simulink model "Vodorod_test_VD"  (R2018b)
settings: Solver=VariableStepAuto  StartTime=0.0  StopTime=1.5  RelTol=1e-3
undefined symbols (not defined in the file): C_cond, DiscIntNeverNeededParam, f, L_dros, L_dros_L4, L_dros_L5, R_cond, R_dros_L4, R_dros_L5, Rc, Rv, Um
libraries: powerlib x26, simulink x2, simulink_extras x1
settings Model: Creator=sr1  LastModifiedBy=sr1

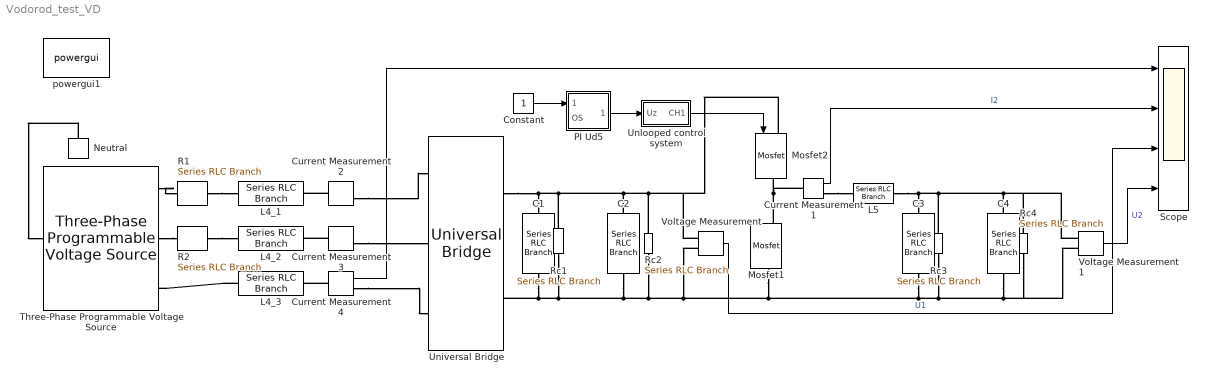
== system Vodorod_test_VD ==
  "C1 " : powerlib/Elements/Series RLC Branch  LConnTagsString=__new0  RConnTagsString=__new0  BranchType=RC  Resistance=R_cond  Inductance=L_dros  SetiL0=off  InitialCurrent=0  Capacitance=C_cond  Setx0=on  InitialVoltage=550  Measurements=None
  C2 : powerlib/Elements/Series RLC Branch  LConnTagsString=__new0  RConnTagsString=__new0  BranchType=RC  Resistance=R_cond  Inductance=L_dros  SetiL0=off  InitialCurrent=0  Capacitance=C_cond  Setx0=on  InitialVoltage=550  Measurements=None
  C3 : powerlib/Elements/Series RLC Branch  LConnTagsString=__new0  RConnTagsString=__new0  BranchType=RC  Resistance=R_cond  Inductance=L_dros  SetiL0=off  InitialCurrent=0  Capacitance=C_cond  Setx0=on  InitialVoltage=0  Measurements=None
  C4 : powerlib/Elements/Series RLC Branch  LConnTagsString=__new0  RConnTagsString=__new0  BranchType=RC  Resistance=R_cond  Inductance=L_dros  SetiL0=off  InitialCurrent=0  Capacitance=C_cond  Setx0=on  InitialVoltage=0  Measurements=None
  Constant : Constant
  Current Measurement{1..4} (4 alike) : powerlib/Measurements/Current Measurement  PhasorSimulation=off  OutputType=Complex  PSBequivalent=0
  "L4_1 " : powerlib/Elements/Series RLC Branch  LConnTagsString=__new0  RConnTagsString=__new0  BranchType=RL  Resistance=R_dros_L4  Inductance=L_dros_L4  SetiL0=off  InitialCurrent=0  Capacitance=1e-6  Setx0=off  InitialVoltage=0  Measurements=None
  "L4_2 " : powerlib/Elements/Series RLC Branch  LConnTagsString=__new0  RConnTagsString=__new0  BranchType=RL  Resistance=R_dros_L4  Inductance=L_dros_L4  SetiL0=off  InitialCurrent=0  Capacitance=1e-6  Setx0=off  InitialVoltage=0  Measurements=None
  "L4_3 " : powerlib/Elements/Series RLC Branch  LConnTagsString=__new0  RConnTagsString=__new0  BranchType=RL  Resistance=R_dros_L4  Inductance=L_dros_L4  SetiL0=off  InitialCurrent=0  Capacitance=1e-6  Setx0=off  InitialVoltage=0  Measurements=None
  "L5 " : powerlib/Elements/Series RLC Branch  LConnTagsString=__new0  RConnTagsString=__new0  BranchType=RL  Resistance=R_dros_L5  Inductance=L_dros_L5  SetiL0=off  InitialCurrent=0  Capacitance=1e-6  Setx0=off  InitialVoltage=0  Measurements=None
  Mosfet1 : powerlib/Power Electronics/Mosfet  Ron=1e-6  Lon=0  Rd=1e-6  Vfd=0  IC=0  Rs=1e5  Cs=inf  Measurements=off
      settings: SourceProductName=Simscape Electrical
  Mosfet2 : powerlib/Power Electronics/Mosfet  Ron=1e-6  Lon=0  Rd=1e-6  Vfd=0  IC=0  Rs=1e5  Cs=inf  Measurements=off
      settings: SourceProductName=Simscape Electrical
  Neutral : powerlib/Elements/Neutral  LConnTagsString=a  NodeNumber=10
      settings: SourceProductName=Simscape Power Systems  SourceProductBaseCode=PS
  PI Ud5 : Subsystem
  R1 : powerlib/Elements/Series RLC Branch  LConnTagsString=__new0  RConnTagsString=__new0  BranchType=R  Resistance=Rv  Inductance=L_dros_L4  SetiL0=off  InitialCurrent=0  Capacitance=1e-6  Setx0=off  InitialVoltage=0  Measurements=None
  R2 : powerlib/Elements/Series RLC Branch  LConnTagsString=__new0  RConnTagsString=__new0  BranchType=R  Resistance=Rv  Inductance=L_dros_L4  SetiL0=off  InitialCurrent=0  Capacitance=1e-6  Setx0=off  InitialVoltage=0  Measurements=None
  Rc{1..4} (4 alike) : powerlib/Elements/Series RLC Branch  LConnTagsString=__new0  RConnTagsString=__new0  BranchType=R  Resistance=Rc  Inductance=L_dros  SetiL0=off  InitialCurrent=0  Capacitance=C_cond  Setx0=off  InitialVoltage=0  Measurements=None
  Scope : Scope  NumInputPorts=4
  Three-Phase Programmable Voltage Source : powerlib/Electrical Sources/Three-Phase Programmable Voltage Source  PositiveSequence=[Um 0 f]  VariationEntity=None  VariationType=Table of time-amplitude pairs  VariationTypeAlt=Step  VariationStep=0.5  VariationRate=10  VariationMagnitude=0.3  VariationFrequency=2  VariationTiming=[1 2]  VariationPhaseA=off  Amplitudes=[1 0.8 1.2 1.0]  TimeValues=[0 0.1 0.15 0.2]  HarmonicGeneration=off  HarmonicA=[3 0.2 -25 0]  HarmonicB=[2 0.15 35 2]  Timing="[0.05  3]"  BusType=swing  Pref=0  Qref=0  Qmin=-inf  Qmax=inf
  Universal Bridge : powerlib/Power Electronics/Universal Bridge  Arms=3  SnubberResistance=1e5  SnubberCapacitance=inf  Device=Diodes  Ron=1e-3  Lon=0  ForwardVoltages="[  0  0  ]"  ForwardVoltage=1  GTOparameters=[ 10e-6 , 20e-6 ]  IGBTparameters=[ 1e-6 , 2e-6 ]  Measurements=None  Measurements_2=None  converterType=Rectifier
  Unlooped control system : Subsystem
  Voltage Measurement : powerlib/Measurements/Voltage Measurement  PhasorSimulation=off  OutputType=Complex  PSBequivalent=0
  Voltage Measurement1 : powerlib/Measurements/Voltage Measurement  PhasorSimulation=off  OutputType=Complex  PSBequivalent=0
  powergui1 : powerlib/powergui  Priority=1  SimulationMode=Discrete  SampleTime=1e-6  frequency=60  Iterations=50  frequencyindice=0  Pbase=100e6  ErrMax=1e-4  UnitsV=kV  UnitsW=MW  buscounter=0  FunctionMessages=off  echomessages=off  EnableUseOfTLC=off  CurrentSourceSwitches=off  DisableSnubberDevices=off  DisableRonSwitches=off  DisableVfSwitches=off  DisplayEquations=off  SolverType=Tustin/Backward Euler (TBE)  Interpol=off  ExternalGateDelay=off  methode=off  Ts=100  x0status=blocks  SPID=off  SwTol=0  HookPort=off  RestoreLinks=warning  ResistiveCurrentMeasurement=off  Frange=[0:2:500]  Ylog=off  Xlog=on  ShowGrid=off  save=off  variable=ZData  structure=0  ZoomFFT=off  StartTime=0.0  cycles=1  DisplayStyle=1  fundamental=60  FreqAxis=off  MaxFrequency=1000  frequencyindicesteady=1  RmsSteady=1  display=off
  wires:
  Current Measurement1/1 -> Scope/2  "I2"
  Voltage Measurement/1 -> Scope/3  "U1"
  Voltage Measurement1/1 -> Scope/4  "U2"
  PI Ud5/1(Out) -> Unlooped control system/1(Uz)
  Constant/1 -> PI Ud5/1(Zad)
  Unlooped control system/1(CH1) -> Mosfet2/1
  Current Measurement4/1 -> Scope/1
  connections:
  "L4_3 "/LConn1 -- Three-Phase Programmable Voltage Source/RConn3
  Neutral/LConn1 -- Three-Phase Programmable Voltage Source/LConn1
  Universal Bridge/RConn1 -- Mosfet2/LConn1 -- Voltage Measurement/LConn1 -- Rc2/LConn1 -- C2/LConn1 -- Rc1/LConn1 -- "C1 "/LConn1
  "C1 "/RConn1 -- Mosfet1/RConn1 -- Voltage Measurement1/LConn2 -- Rc4/RConn1 -- C4/RConn1 -- Rc3/RConn1 -- C3/RConn1 -- Voltage Measurement/LConn2 -- Rc2/RConn1 -- C2/RConn1 -- Rc1/RConn1 -- Universal Bridge/RConn2
  "L5 "/RConn1 -- Voltage Measurement1/LConn1 -- Rc4/LConn1 -- C4/LConn1 -- Rc3/LConn1 -- C3/LConn1
  Current Measurement1/RConn1 -- "L5 "/LConn1
  Three-Phase Programmable Voltage Source/RConn1 -- R1/LConn1
  Three-Phase Programmable Voltage Source/RConn2 -- R2/LConn1
  Current Measurement2/LConn1 -- "L4_1 "/RConn1
  Current Measurement2/RConn1 -- Universal Bridge/LConn1
  Current Measurement3/LConn1 -- "L4_2 "/RConn1
  Current Measurement3/RConn1 -- Universal Bridge/LConn2
  Current Measurement4/LConn1 -- "L4_3 "/RConn1
  Current Measurement4/RConn1 -- Universal Bridge/LConn3
  Mosfet1/LConn1 -- Current Measurement1/LConn1 -- Mosfet2/RConn1
  R1/RConn1 -- "L4_1 "/LConn1
  R2/RConn1 -- "L4_2 "/LConn1

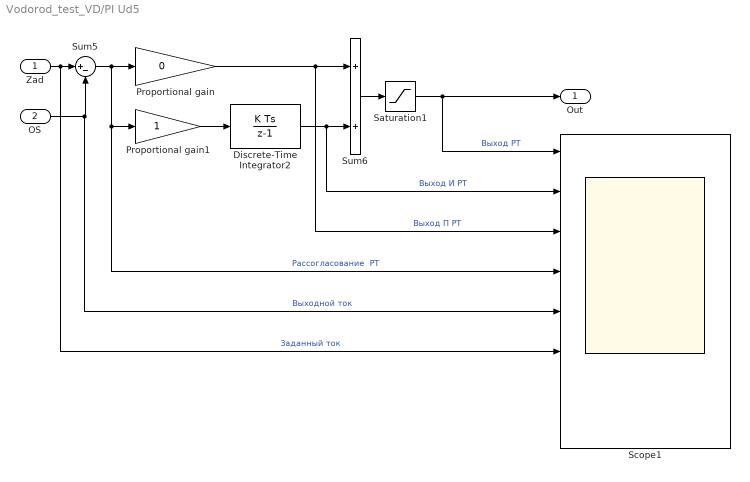
== system Vodorod_test_VD/PI Ud5 ==
  Zad : Inport
  OS : Inport  Port=2
  Discrete-Time Integrator2 : DiscreteIntegrator  SampleTime=-1  LimitOutput=on  UpperSaturationLimit=1  LowerSaturationLimit=0  ICPrevOutput=DiscIntNeverNeededParam  ICPrevScaledInput=DiscIntNeverNeededParam
  Proportional gain : Gain  Gain=0  SaturateOnIntegerOverflow=on  OutDataTypeStr=Inherit: Same as input  ParamDataTypeStr=Inherit: Same as input
  Proportional gain1 : Gain  SaturateOnIntegerOverflow=on  OutDataTypeStr=Inherit: Same as input  ParamDataTypeStr=Inherit: Same as input
  Saturation1 : Saturate  UpperLimit=1  LowerLimit=0
  Scope1 : Scope  NumInputPorts=8
  Sum5 : Sum  Inputs=|+-  SaturateOnIntegerOverflow=on  InputSameDT=on  OutDataTypeStr=Inherit: Same as first input
  Sum6 : Sum  SaturateOnIntegerOverflow=on  InputSameDT=on  OutDataTypeStr=Inherit: Same as first input
  Out : Outport
  wires:
  Proportional gain/1 -> Scope1/3, Sum6/1  "Выход П РТ"
  Discrete-Time Integrator2/1 -> Sum6/2, Scope1/2  "Выход И РТ"
  OS/1 -> Scope1/5, Sum5/2  "Выходной ток"
  Zad/1 -> Scope1/6, Sum5/1  "Заданный ток"
  Sum5/1 -> Proportional gain1/1, Scope1/4, Proportional gain/1  "Рассогласование  РТ"
  Sum6/1 -> Saturation1/1
  Saturation1/1 -> Out/1, Scope1/1  "Выход РТ"
  Proportional gain1/1 -> Discrete-Time Integrator2/1

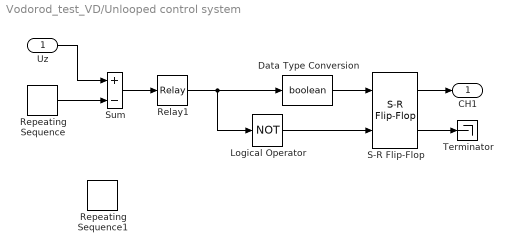
== system Vodorod_test_VD/Unlooped control system ==
  Uz : Inport
  Data Type Conversion : DataTypeConversion  OutDataTypeStr=boolean
  Logical Operator : Logic  Operator=NOT  AllPortsSameDT=off  OutDataTypeStr=boolean
  Relay1 : Relay  OnSwitchValue=0.01  OffSwitchValue=-0.01
  Repeating Sequence : simulink/Sources/Repeating Sequence  rep_seq_t=[0 0.00025]  rep_seq_y=[0 1]
  Repeating Sequence1 : simulink/Sources/Repeating Sequence  rep_seq_t="[0  0.000125 0.00025]"  rep_seq_y=[0 1 0]
  S-R Flip-Flop : simulink_extras/Flip Flops/S-R Flip-Flop  initial_condition=0
  Sum : Sum  Inputs=+-
  Terminator : Terminator
  CH1 : Outport
  wires:
  S-R Flip-Flop/1 -> CH1/1
  Data Type Conversion/1 -> S-R Flip-Flop/1
  Logical Operator/1 -> S-R Flip-Flop/2
  Relay1/1 -> Logical Operator/1, Data Type Conversion/1
  Repeating Sequence/1 -> Sum/2
  Uz/1 -> Sum/1
  Sum/1 -> Relay1/1
  S-R Flip-Flop/2 -> Terminator/1
